simulink model "asynchron"  (R2017a)
settings: Solver=VariableStepAuto  StartTime=0.0  StopTime=100  RelTol=1e-3
libraries: simulink x1
settings Model: Creator=johan  LastModifiedBy=johan

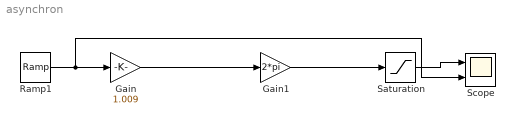
== system asynchron ==
  Gain : Gain  Gain=1.009
  Gain1 : Gain  Gain=2*pi
  Ramp1 : simulink/Sources/Ramp  slope=1  start=0  X0=0
  Saturation : Saturate  UpperLimit=317  LowerLimit=0
  Scope : Scope  NumInputPorts=2
  wires:
  Gain/1 -> Gain1/1
  Gain1/1 -> Saturation/1
  Saturation/1 -> Scope/1
  Ramp1/1 -> Scope/2, Gain/1
